simulink model "Aerodynamic_and_gravity_Forces"  (R2013a)
settings: Solver=ode45  StartTime=0.0  StopTime=10.0  RelTol=1e-3
values from neighbouring files (symbols this model uses):
  b_w = 21.94    [Donee.m]
  C = 9.55    [Donee.m]
  S_w = (Cr_w + Ct_w)*b_w/4    (= 95.762615)    [Donee.m]
settings Model: Creator=Ibrahim_B92  LastModifiedBy=Ibrahim_B92

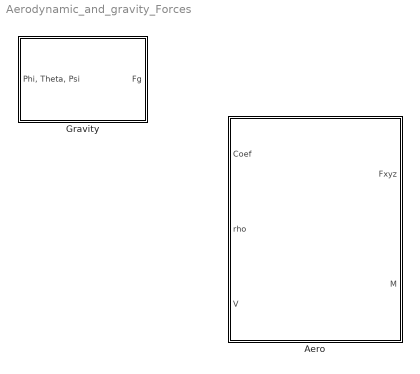
== system Aerodynamic_and_gravity_Forces ==
  "Aero " : Subsystem
  Gravity : Subsystem

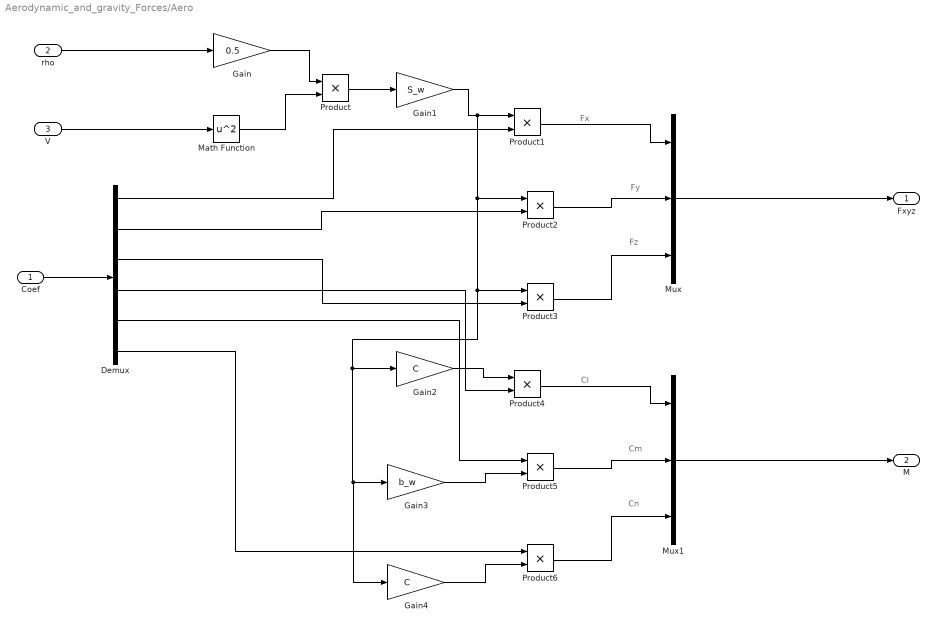
== system Aerodynamic_and_gravity_Forces/Aero  ==
  note: Fz
  note: Fy
  note: Fx
  note: Cn
  note: Cm
  note: Cl
  Coef : Inport
  rho : Inport  Port=2
  V : Inport  Port=3
  Demux : Demux  Outputs=6
  Gain : Gain  Gain=0.5
  Gain1 : Gain  Gain=S_w
  Gain2 : Gain  Gain=C
  Gain3 : Gain  Gain=b_w
  Gain4 : Gain  Gain=C
  Math Function : Math  Operator=square  SaturateOnIntegerOverflow=on
  Mux : Mux  Inputs=3
  Mux1 : Mux  Inputs=3
  Product{,1..6} (7 alike) : Product
  Fxyz : Outport
  M : Outport  Port=2
  wires:
  rho/1 -> Gain/1
  V/1 -> Math Function/1
  Math Function/1 -> Product/2
  Gain/1 -> Product/1
  Product/1 -> Gain1/1
  Coef/1 -> Demux/1
  Demux/1 -> Product1/2
  Gain1/1 -> Gain4/1, Gain3/1, Gain2/1, Product3/1, Product2/1, Product1/1
  Product1/1 -> Mux/1
  Demux/2 -> Product2/2
  Product2/1 -> Mux/2
  Demux/3 -> Product3/2
  Product3/1 -> Mux/3
  Product4/1 -> Mux1/1
  Product5/1 -> Mux1/2
  Product6/1 -> Mux1/3
  Gain2/1 -> Product4/1
  Demux/4 -> Product4/2
  Gain3/1 -> Product5/2
  Demux/5 -> Product5/1
  Gain4/1 -> Product6/2
  Demux/6 -> Product6/1
  Mux1/1 -> M/1
  Mux/1 -> Fxyz/1

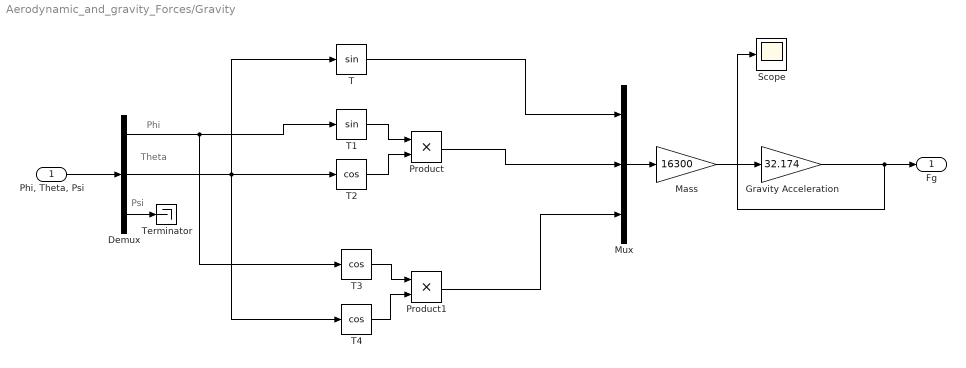
== system Aerodynamic_and_gravity_Forces/Gravity ==
  note: Psi
  note: Theta
  note: Phi
  "Phi, Theta, Psi" : Inport
  Demux : Demux  Outputs=3
  Gravity Acceleration : Gain  Gain=32.174
  Mass : Gain  Gain=16300
  Mux : Mux  Inputs=3
  Product : Product
  Product1 : Product
  Scope : Scope
      settings: SaveName=ScopeData6
  T : Trigonometry
  T1 : Trigonometry
  T2 : Trigonometry  Operator=cos
  T3 : Trigonometry  Operator=cos
  T4 : Trigonometry  Operator=cos
  Terminator : Terminator
  Fg : Outport
  wires:
  T3/1 -> Product1/1
  T4/1 -> Product1/2
  T1/1 -> Product/1
  T2/1 -> Product/2
  "Phi, Theta, Psi"/1 -> Demux/1
  Demux/2 -> T4/1, T2/1, T/1
  Demux/1 -> T3/1, T1/1
  Demux/3 -> Terminator/1
  T/1 -> Mux/1
  Product/1 -> Mux/2
  Product1/1 -> Mux/3
  Mux/1 -> Mass/1
  Mass/1 -> Gravity Acceleration/1
  Gravity Acceleration/1 -> Scope/1, Fg/1
